simulink model "model_InputConditioningAutoStop_Test"  (R2024a)
settings: Solver=VariableStepAuto  StartTime=0.0  StopTime=10.0  RelTol=1e-3
settings Model: Creator=Gabriel  LastModifiedBy=Gabriel

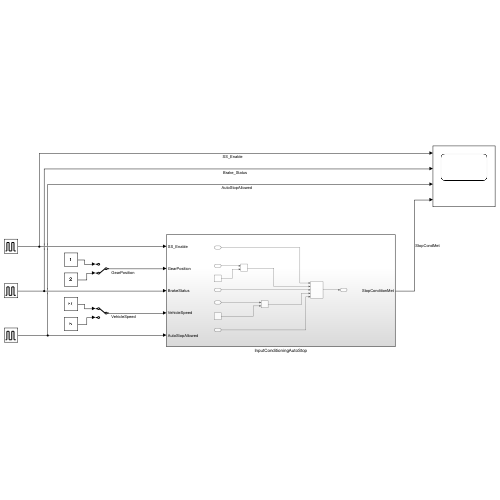
[thumbnail: Simulink's stored preview of the top-level diagram]
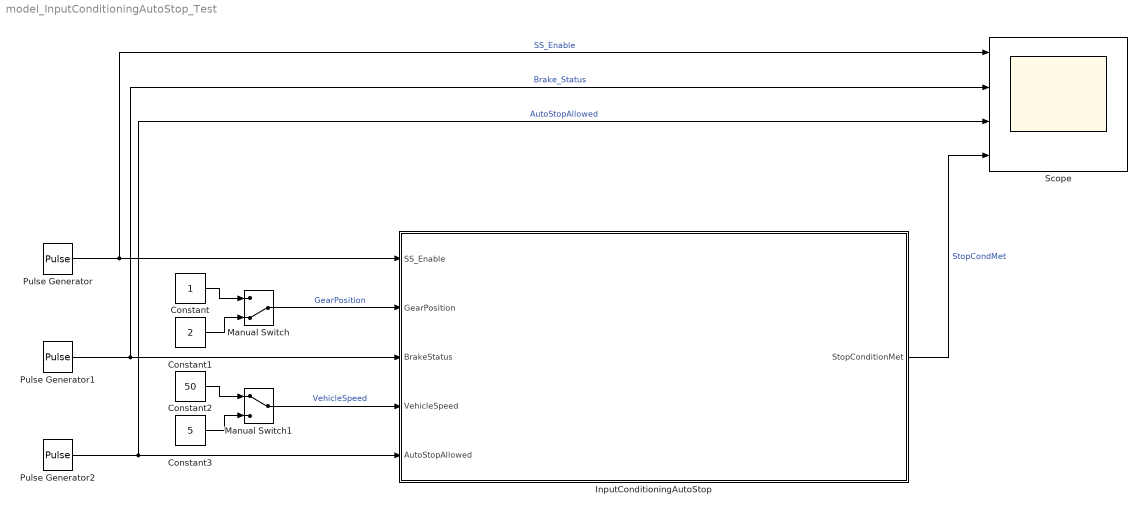
== system model_InputConditioningAutoStop_Test ==
  Constant : Constant
  Constant1 : Constant  Value=2
  Constant2 : Constant  Value=50
  Constant3 : Constant  Value=5
  InputConditioningAutoStop : Subsystem
  Manual Switch : ManualSwitch  CurrentSetting=0
  Manual Switch1 : ManualSwitch
  Pulse Generator : DiscretePulseGenerator  PulseType=Time based  PulseWidth=50
  Pulse Generator1 : DiscretePulseGenerator  PulseType=Time based  PulseWidth=30
  Pulse Generator2 : DiscretePulseGenerator  PulseType=Time based  PulseWidth=60
  Scope : Scope  NumInputPorts=4
  wires:
  Pulse Generator/1 -> Scope/1, InputConditioningAutoStop/1(SS_Enable)  "SS_Enable"
  Pulse Generator1/1 -> Scope/2, InputConditioningAutoStop/3(BrakeStatus)  "Brake_Status"
  Pulse Generator2/1 -> Scope/3, InputConditioningAutoStop/5(AutoStopAllowed)  "AutoStopAllowed"
  Constant/1 -> Manual Switch/1
  Constant1/1 -> Manual Switch/2
  Manual Switch/1 -> InputConditioningAutoStop/2(GearPosition)  "GearPosition"
  Constant3/1 -> Manual Switch1/2
  Constant2/1 -> Manual Switch1/1
  Manual Switch1/1 -> InputConditioningAutoStop/4(VehicleSpeed)  "VehicleSpeed"
  InputConditioningAutoStop/1(StopConditionMet) -> Scope/4  "StopCondMet"

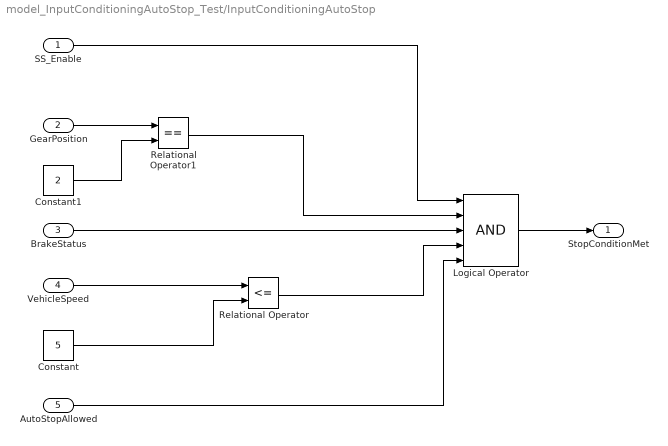
== system model_InputConditioningAutoStop_Test/InputConditioningAutoStop ==
  SS_Enable : Inport
  GearPosition : Inport  Port=2
  BrakeStatus : Inport  Port=3
  VehicleSpeed : Inport  Port=4
  AutoStopAllowed : Inport  Port=5
  Constant : Constant  Value=5
  Constant1 : Constant  Value=2
  Logical Operator : Logic  Inputs=5  AllPortsSameDT=off  OutDataTypeStr=boolean
  Relational Operator : RelationalOperator  Operator=<=  OutDataTypeStr=boolean  RndMeth=Simplest  InputSameDT=off
  Relational Operator1 : RelationalOperator  Operator===  OutDataTypeStr=boolean  RndMeth=Simplest  InputSameDT=off
  StopConditionMet : Outport
  wires:
  VehicleSpeed/1 -> Relational Operator/1
  Constant/1 -> Relational Operator/2
  SS_Enable/1 -> Logical Operator/1
  Relational Operator/1 -> Logical Operator/4
  AutoStopAllowed/1 -> Logical Operator/5
  GearPosition/1 -> Relational Operator1/1
  Relational Operator1/1 -> Logical Operator/2
  BrakeStatus/1 -> Logical Operator/3
  Constant1/1 -> Relational Operator1/2
  Logical Operator/1 -> StopConditionMet/1
